simulink model "virtualbus_0002_pass"  (R2020a)
settings: Solver=VariableStepAuto  StartTime=0.0  StopTime=10.0  RelTol=1e-3
settings Model: DataDictionary=correct_types.sldd  Creator=raarenst  LastModifiedBy=raarenst
settings DebuggingCC: UnconnectedInputMsg=none  UnconnectedOutputMsg=none  UnconnectedLineMsg=none
settings ModelReferenceCC: EnableRefExpFcnMdlSchedulingChecks=off
settings RTWCC: Description=Generic Real-Time Target

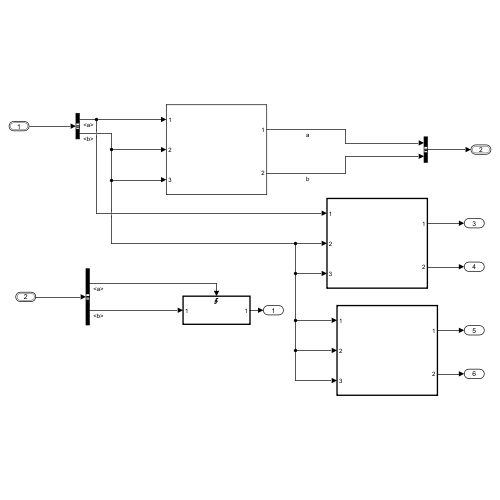
[thumbnail: Simulink's stored preview of the top-level diagram]
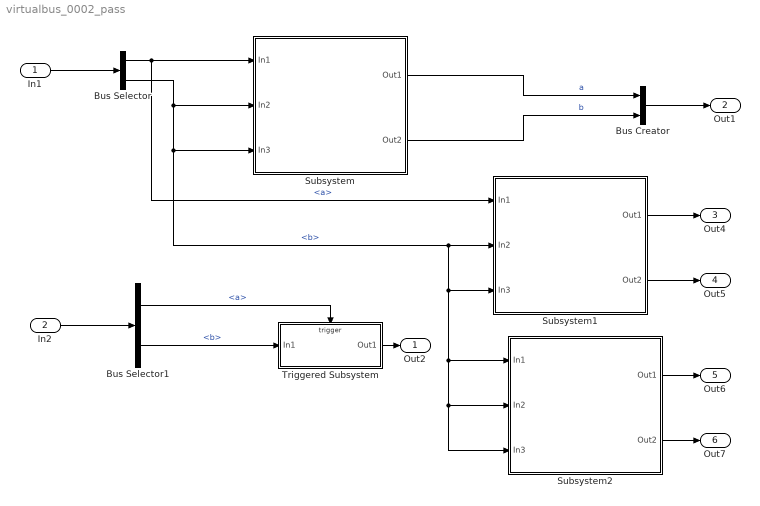
== system virtualbus_0002_pass ==
  In1 : Inport  OutDataTypeStr=Bus: BusObject
  In2 : Inport  Port=2  OutDataTypeStr=Bus: BusObject
  Bus Creator : BusCreator  Inputs=2  OutDataTypeStr=Bus: BusObject
  Bus Selector : BusSelector  OutputSignals=a,b
  Bus Selector1 : BusSelector  OutputSignals=a,b
  Subsystem : Subsystem
  Subsystem1 : Subsystem  TreatAsAtomicUnit=on
  Subsystem2 : Subsystem  TreatAsAtomicUnit=on  mask{Parameter1=on}
  Triggered Subsystem : Subsystem  TreatAsAtomicUnit=on
  Out2 : Outport
  Out1 : Outport  Port=2  OutDataTypeStr=Bus: BusObject
  Out4 : Outport  Port=3
  Out5 : Outport  Port=4
  Out6 : Outport  Port=5
  Out7 : Outport  Port=6
  wires:
  Bus Selector/1 -> Subsystem1/1(In1), Subsystem/1(In1)  "<a>"
  Triggered Subsystem/1(Out1) -> Out2/1
  Bus Selector1/2 -> Triggered Subsystem/1(In1)  "<b>"
  Bus Selector1/1 -> Triggered Subsystem/Trigger  "<a>"
  Bus Selector/2 -> Subsystem1/3(In3), Subsystem2/1(In1), Subsystem2/2(In2), Subsystem2/3(In3), Subsystem1/2(In2), Subsystem/3(In3), Subsystem/2(In2)  "<b>"
  Subsystem/1(Out1) -> Bus Creator/1  "a"
  Subsystem/2(Out2) -> Bus Creator/2  "b"
  Subsystem1/1(Out1) -> Out4/1
  Subsystem1/2(Out2) -> Out5/1
  Subsystem2/1(Out1) -> Out6/1
  Subsystem2/2(Out2) -> Out7/1
  In1/1 -> Bus Selector/1
  Bus Creator/1 -> Out1/1
  In2/1 -> Bus Selector1/1

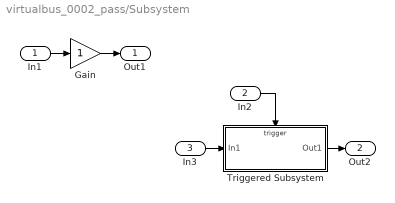
== system virtualbus_0002_pass/Subsystem ==
  In1 : Inport
  In2 : Inport  Port=2
  In3 : Inport  Port=3
  Gain : Gain
  Triggered Subsystem : Subsystem  TreatAsAtomicUnit=on
  Out1 : Outport
  Out2 : Outport  Port=2
  wires:
  In3/1 -> Triggered Subsystem/1(In1)
  In1/1 -> Gain/1
  In2/1 -> Triggered Subsystem/Trigger
  Gain/1 -> Out1/1
  Triggered Subsystem/1(Out1) -> Out2/1

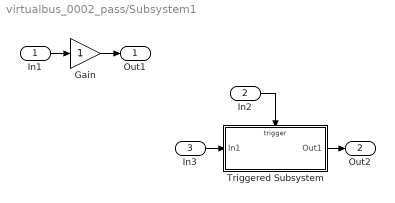
== system virtualbus_0002_pass/Subsystem1 ==
  In1 : Inport
  In2 : Inport  Port=2
  In3 : Inport  Port=3
  Gain : Gain
  Triggered Subsystem : Subsystem  TreatAsAtomicUnit=on
  Out1 : Outport
  Out2 : Outport  Port=2
  wires:
  Triggered Subsystem/1(Out1) -> Out2/1
  Gain/1 -> Out1/1
  In2/1 -> Triggered Subsystem/Trigger
  In1/1 -> Gain/1
  In3/1 -> Triggered Subsystem/1(In1)

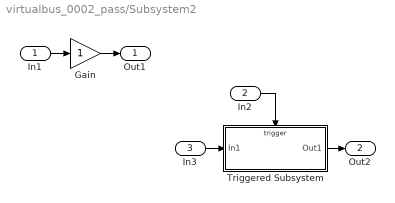
== system virtualbus_0002_pass/Subsystem2 ==
  In1 : Inport
  In2 : Inport  Port=2
  In3 : Inport  Port=3
  Gain : Gain
  Triggered Subsystem : Subsystem  TreatAsAtomicUnit=on
  Out1 : Outport
  Out2 : Outport  Port=2
  wires:
  In3/1 -> Triggered Subsystem/1(In1)
  In1/1 -> Gain/1
  In2/1 -> Triggered Subsystem/Trigger
  Gain/1 -> Out1/1
  Triggered Subsystem/1(Out1) -> Out2/1

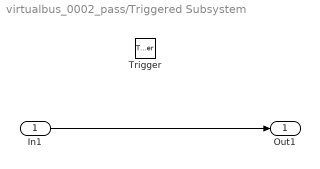
== system virtualbus_0002_pass/Triggered Subsystem ==
  In1 : Inport
  Trigger : TriggerPort  VariantControl=(inherit)
  Out1 : Outport
  wires:
  In1/1 -> Out1/1

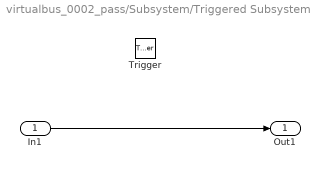
== system virtualbus_0002_pass/Subsystem/Triggered Subsystem ==
  In1 : Inport
  Trigger : TriggerPort  VariantControl=(inherit)
  Out1 : Outport
  wires:
  In1/1 -> Out1/1

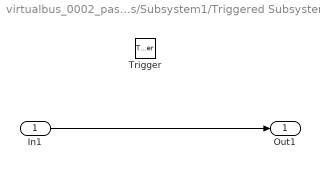
== system virtualbus_0002_pass/Subsystem1/Triggered Subsystem ==
  In1 : Inport
  Trigger : TriggerPort  VariantControl=(inherit)
  Out1 : Outport
  wires:
  In1/1 -> Out1/1

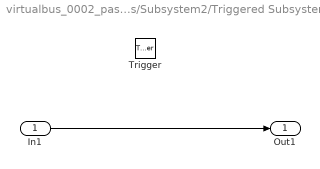
== system virtualbus_0002_pass/Subsystem2/Triggered Subsystem ==
  In1 : Inport
  Trigger : TriggerPort  VariantControl=(inherit)
  Out1 : Outport
  wires:
  In1/1 -> Out1/1
